simulink model "sun_traking_system_model"  (R2020b)
settings: Solver=VariableStepAuto  StartTime=0.0  StopTime=15*3600  RelTol=1e-3
undefined symbols (not defined in the file): J, Kd, Kf, Kg, Kt, L, R
libraries: pid_lib x1
settings Model: Creator=s023793  LastModifiedBy=s023793
settings DataIOCC: ExternalInput=[sunTime sunPosition]  LoadExternalInput=on

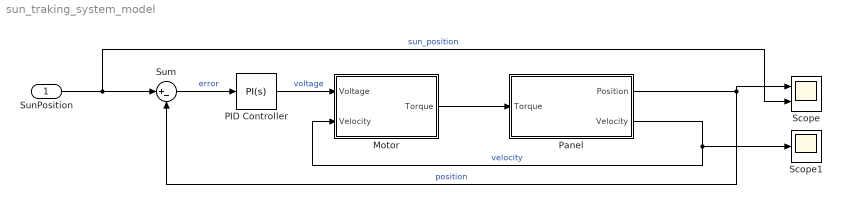
== system sun_traking_system_model ==
  SunPosition : Inport
  Motor : Subsystem
  PID Controller : pid_lib/PID Controller  Controller=PI  Form=Parallel  TimeDomain=Continuous-time  UseExternalTs=off  SampleTime=-1  IntegratorMethod=Forward Euler  FilterMethod=Forward Euler  ControllerParametersSource=internal  P=240  I=180  D=0  UseFilter=on  N=0.000690730423360061  TunerSelectOption=Transfer Function Based (PID Tuner App)  InitialConditionSource=internal  InitialConditionForIntegrator=0  InitialConditionForFilter=0  DifferentiatorICPrevScaledInput=0  ExternalReset=none  TrackingMode=off  Kt=1  LimitOutput=off  SatLimitsSource=internal  UpperSaturationLimit=inf  LowerSaturationLimit=-inf  LinearizeAsGain=on  AntiWindupMode=none  Kb=1  POutMin=[]  POutMax=[]  IOutMin=[]  IOutMax=[]  DOutMin=[]  DOutMax=[]  NOutMin=[]  NOutMax=[]  SumOutMin=[]  SumOutMax=[]  SaturationOutMin=[]  SaturationOutMax=[]  PParamMin=[]  PParamMax=[]  IParamMin=[]  IParamMax=[]  DParamMin=[]  DParamMax=[]  NParamMin=[]  NParamMax=[]  KbParamMin=[]  KbParamMax=[]  KtParamMin=[]  KtParamMax=[]  KbOutMin=[]  KbOutMax=[]  KtOutMin=[]  KtOutMax=[]  IntegratorOutMin=[]  IntegratorOutMax=[]  FilterOutMin=[]  FilterOutMax=[]  SumI1OutMin=[]  SumI1OutMax=[]  SumI2OutMin=[]  SumI2OutMax=[]  SumI3OutMin=[]  SumI3OutMax=[]  SumI4OutMin=[]  SumI4OutMax=[]  SumDOutMin=[]  SumDOutMax=[]  DifferentiatorOutMin=[]  DifferentiatorOutMax=[]  FilterDiffOutCoefMin=[]  FilterDiffOutCoefMax=[]  ReciprocalOutMin=[]  ReciprocalOutMax=[]  SumDenOutMin=[]  SumDenOutMax=[]  SumNumOutMin=[]  SumNumOutMax=[]  DivideOutMin=[]  DivideOutMax=[]  UdiffTsProdOutMin=[]  UdiffTsProdOutMax=[]  NTsProdOutMin=[]  NTsProdOutMax=[]  UintegralTsProdOutMin=[]  UintegralTsProdOutMax=[]  UngainTsProdOutMin=[]  UngainTsProdOutMax=[]  IntegratorContinuousStateAttributes=''  IntegratorStateMustResolveToSignalObject=off  IntegratorRTWStateStorageClass=Auto  FilterContinuousStateAttributes=''  FilterStateMustResolveToSignalObject=off  FilterRTWStateStorageClass=Auto  ParallelPVariant=InternalParameters  IdealPVariant=Disabled  IVariant=InternalParameters  DVariant=Disabled  IntegratorVariant=Continuous  SatVariant=Disabled  AWVariant=Passthrough  PCopyVariant=Disabled  TRVariant=Disabled  FdbkBlocksVariant=Forward  IdealPFdbkVariant=Disabled  SatFdbkVariant=Disabled  DerivativeFilterVariant=Disabled  NVariant=Disabled  NCopyVariant=Disabled_SignalSpec  FilterICVariant=Disabled  IntegratorICVariant=InternalICs  ExternalResetVariant=Disabled  TRSumVariant=Passthrough  SumFdbkVariant=Disabled  SumVariant=Sum_PI  TsampFilterVariant=InternalTs  TsampNgainVariant=Passthrough  TsampIntegralVariant=Passthrough  ExternalSaturationOutDataTypeStr=Inherit: Same as second input
  Panel : Subsystem
  Scope : Scope  NumInputPorts=2
  Scope1 : Scope
  Sum : Sum  Inputs=|+-
  wires:
  Panel/1(Position) -> Sum/2, Scope/1  "position"
  Panel/2(Velocity) -> Motor/2(Velocity), Scope1/1  "velocity"
  PID Controller/1 -> Motor/1(Voltage)  "voltage"
  Motor/1(Torque) -> Panel/1(Torque)
  SunPosition/1 -> Scope/2, Sum/1  "sun_position"
  Sum/1 -> PID Controller/1  "error"

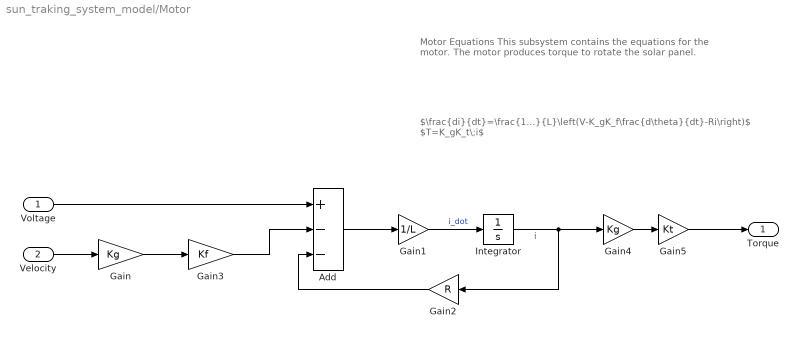
== system sun_traking_system_model/Motor ==
  note: i
  note: $\frac{di}{dt}=\frac{1}{L}\left(V-K_gK_f\frac{d\theta}{dt}-Ri\right)$
      | $T=K_gK_t\;i$
  note: Motor Equations
      |
      | This subsystem contains the equations for the motor. The motor produces torque to rotate the solar panel.
  Voltage : Inport
  Velocity : Inport  Port=2
  Add : Sum  Inputs=+--
  Gain : Gain  Gain=Kg
  Gain1 : Gain  Gain=1/L
  Gain2 : Gain  Gain=R
  Gain3 : Gain  Gain=Kf
  Gain4 : Gain  Gain=Kg
  Gain5 : Gain  Gain=Kt
  Integrator : Integrator
  Torque : Outport
  wires:
  Integrator/1 -> Gain4/1, Gain2/1
  Velocity/1 -> Gain/1
  Voltage/1 -> Add/1
  Add/1 -> Gain1/1
  Gain2/1 -> Add/3
  Gain1/1 -> Integrator/1  "i_dot"
  Gain/1 -> Gain3/1
  Gain3/1 -> Add/2
  Gain4/1 -> Gain5/1
  Gain5/1 -> Torque/1

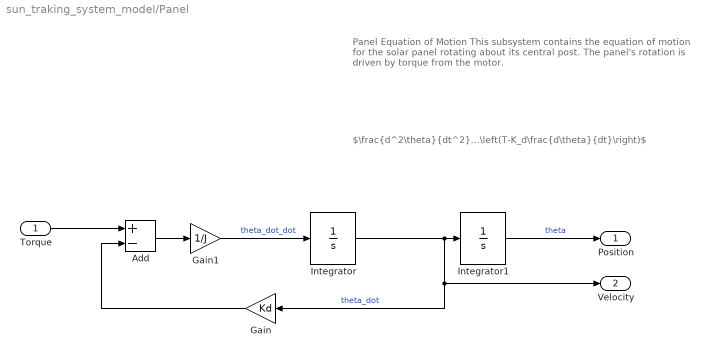
== system sun_traking_system_model/Panel ==
  note: $\frac{d^2\theta}{dt^2}=\frac{1}{J}\left(T-K_d\frac{d\theta}{dt}\right)$
  note: Panel Equation of Motion
      |
      | This subsystem contains the equation of motion for the solar panel rotating about its central post. The panel's rotation is driven by torque from the motor.
  Torque : Inport
  Add : Sum  Inputs=+-
  Gain : Gain  Gain=Kd
  Gain1 : Gain  Gain=1/J
  Integrator : Integrator
  Integrator1 : Integrator
  Position : Outport
  Velocity : Outport  Port=2
  wires:
  Integrator1/1 -> Position/1  "theta"
  Gain1/1 -> Integrator/1  "theta_dot_dot"
  Gain/1 -> Add/2
  Integrator/1 -> Integrator1/1, Velocity/1, Gain/1  "theta_dot"
  Torque/1 -> Add/1
  Add/1 -> Gain1/1
